simulink model "StanfordArm"  (Simulink 7.6)
settings: Solver=ode45  StartTime=0.0  StopTime=10.0  RelTol=1e-3
libraries: roblocks x3, simulink x1
settings Model: Creator=mahyar  LastModifiedBy=mahyar

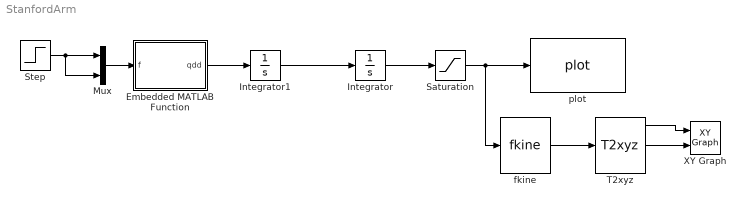
== system StanfordArm ==
  Embedded MATLAB Function : Stateflow chart  TreatAsAtomicUnit=on
  Integrator : Integrator
  Integrator1 : Integrator
  Mux : Mux  Inputs=2
  Saturation : Saturate  UpperLimit=2  LowerLimit=-2
  Step : Step  After=-1  SampleTime=0
  T2xyz : roblocks/T2xyz  SystemSampleTime=-1
  XY Graph : simulink/Sinks/XY Graph  SystemSampleTime=-1  xmin=-2  xmax=2  ymin=-2  ymax=2  st=-1
  fkine : roblocks/fkine  SystemSampleTime=-1  robot=r
  plot : roblocks/plot  SystemSampleTime=-1  robot=r
  wires:
  Mux/1 -> Embedded MATLAB Function/1(f)
  Step/1 -> Mux/1, Mux/2
  Embedded MATLAB Function/1(qdd) -> Integrator1/1
  Integrator1/1 -> Integrator/1
  Integrator/1 -> Saturation/1
  Saturation/1 -> plot/1, fkine/1
  fkine/1 -> T2xyz/1
  T2xyz/1 -> XY Graph/1
  T2xyz/2 -> XY Graph/2

== matlab function Embedded MATLAB Function ==
  data: f input double; qdd output double
function qdd = fcn(f)

m1 = 1;
m2 = 1;
g = 9.8;

qdd1=-(1/(m1+m2))*(f(1)-g*(m1+m2));
qdd2=(1/m2)*(f(2))
qdd = [qdd1;qdd2];
